simulink model "Modelo_Respiratorio"  (R2018a)
settings: Solver=FixedStepAuto  StartTime=0.0  StopTime=15  FixedStep=0.01  MaxStep=0.05  RelTol=1e-3  AbsTol=1e-3
model workspace (MAT data in the model file):
  FR = Simulink.Parameter
  FR.Value = Simulink.data.Expression
  FR.Value.ExpressionString = "FR"
  FR.DataType = 'auto'
  FR.Dimensions = -1
values from neighbouring files (symbols this model uses):
  a = str2num(get(handles.FR, 'String'))    [Ventiladorcito.m]
  b = str2num(get(handles.PEEP, 'String'))    [Ventiladorcito.m]
  c = str2num(get(handles.PP, 'String'))    [Ventiladorcito.m]
  d = round(1/(d+1),2)*100    [Ventiladorcito.m]
  f = str2num(get(handles.CL, 'String'))    [Ventiladorcito.m]
  g = str2num(get(handles.Cw, 'String'))    [Ventiladorcito.m]
  h = str2num(get(handles.Rc, 'String'))    [Ventiladorcito.m]
  j = str2num(get(handles.Rp, 'String'))    [Ventiladorcito.m]
  k = str2num(get(handles.Cs, 'String'))    [Ventiladorcito.m]
settings Model: Creator=Biomecanica  LastModifiedBy=David
settings SolverCC: AutoScaleAbsTol=off
settings DataIOCC: SaveFormat=Array  SignalLoggingSaveFormat=ModelDataLogs  SaveOutput=off  SaveTime=off
settings OptimizationCC: BlockReduction=off  BooleanDataType=off  LifeSpan=inf
settings DebuggingCC: SaveWithParameterizedLinksMsg=none  UnderspecifiedInitializationDetection=Classic  MergeDetectMultiDrivingBlocksExec=none  SignalResolutionControl=TryResolveAllWithWarning  MultiTaskDSMMsg=warning  MultiTaskCondExecSysMsg=none  SFUnexpectedBacktrackingDiag=warning  SFNoUnconditionalDefaultTransitionDiag=warning  SFExecutionAtInitializationDiag=none
settings HardwareCC: TargetUnknown=on
settings ModelReferenceCC: PropagateSignalLabelsOutOfModel=off
settings RTWCC: TemplateMakefile=grt_vc.tmf
settings CodeAppCC: StateflowObjectComments=on
settings GRTTargetCC: TargetLangStandard=C89/C90 (ANSI)  CombineOutputUpdateFcns=off  GRTInterface=on
settings ConfigComp: CovMetricSettings=dw  CovHtmlReporting=on  CovSaveCumulativeToWorkspaceVar=on  CovSaveSingleToWorkspaceVar=on  CovExternalEMLEnable=off

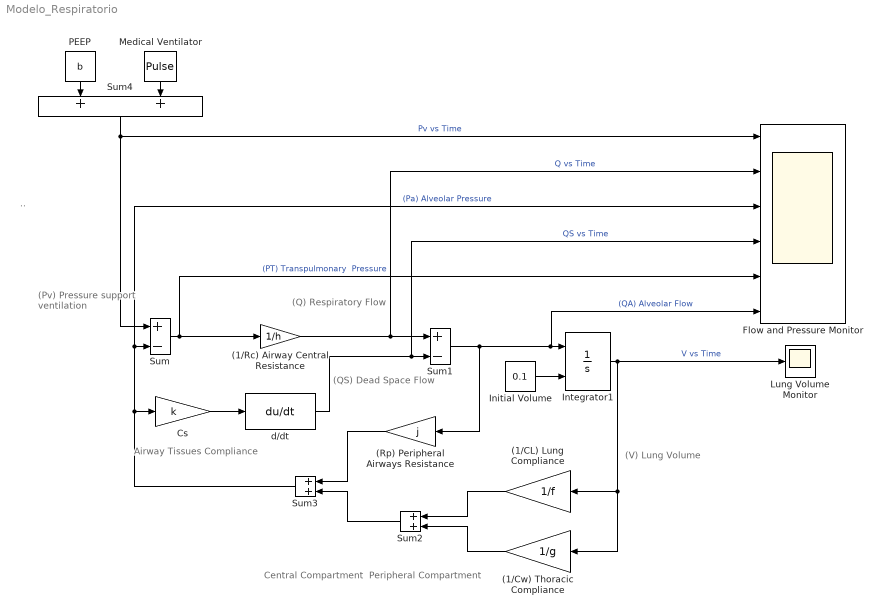
== system Modelo_Respiratorio ==
  note: Airway Tissues
      | Compliance
  note: ..
  note: Peripheral
      | Compartment
  note: (Pv)
      | Pressure support ventilation
  note: (Q)
      | Respiratory
      | Flow
  note: (V)
      | Lung Volume
  note: (QS)
      | Dead Space
      | Flow
  note: Central
      | Compartment
  " Medical Ventilator" : DiscretePulseGenerator  PulseType=Time based  Amplitude=c  Period=60/a  PulseWidth=d
  (1/CL) Lung Compliance : Gain  Gain=1/f  SaturateOnIntegerOverflow=on  OutDataTypeStr=Inherit: Same as input  ParamDataTypeStr=Inherit: Same as input
  (1/Cw) Thoracic Compliance : Gain  Gain=1/g  SaturateOnIntegerOverflow=on  OutDataTypeStr=Inherit: Same as input  ParamDataTypeStr=Inherit: Same as input
  "(1/Rc) Airway Central Resistance " : Gain  Gain=1/h  SaturateOnIntegerOverflow=on  OutDataTypeStr=Inherit: Same as input  ParamDataTypeStr=Inherit: Same as input
  "(Rp) Peripheral Airways Resistance " : Gain  Gain=j  SaturateOnIntegerOverflow=on  OutDataTypeStr=Inherit: Same as input  ParamDataTypeStr=Inherit: Same as input
  "Cs " : Gain  Gain=k  SaturateOnIntegerOverflow=on  OutDataTypeStr=Inherit: Same as input  ParamDataTypeStr=Inherit: Same as input
  Flow and Pressure Monitor : Scope  NumInputPorts=6
  Initial Volume : Constant  Value=0.1
  Integrator1 : Integrator  InitialConditionSource=external
  Lung Volume Monitor : Scope
  PEEP : Constant  Value=b
  Sum : Sum  Inputs=+-  SaturateOnIntegerOverflow=on  InputSameDT=on  OutDataTypeStr=Inherit: Same as first input
  Sum1 : Sum  Inputs=+-  SaturateOnIntegerOverflow=on  InputSameDT=on  OutDataTypeStr=Inherit: Same as first input
  Sum2 : Sum  SaturateOnIntegerOverflow=on  InputSameDT=on  OutDataTypeStr=Inherit: Same as first input
  Sum3 : Sum  SaturateOnIntegerOverflow=on  InputSameDT=on  OutDataTypeStr=Inherit: Same as first input
  Sum4 : Sum  SaturateOnIntegerOverflow=on  InputSameDT=on  OutDataTypeStr=Inherit: Same as first input
  "d/dt " : Derivative  CoefficientInTFapproximation=1
  wires:
  Sum/1 -> "(1/Rc) Airway Central Resistance "/1, Flow and Pressure Monitor/5  "(PT) Transpulmonary  Pressure"
  "(1/Rc) Airway Central Resistance "/1 -> Sum1/1, Flow and Pressure Monitor/2  "Q vs Time"
  "Cs "/1 -> "d/dt "/1
  "d/dt "/1 -> Flow and Pressure Monitor/4, Sum1/2  "QS vs Time"
  (1/CL) Lung Compliance/1 -> Sum2/1
  (1/Cw) Thoracic Compliance/1 -> Sum2/2
  Integrator1/1 -> Lung Volume Monitor/1, (1/CL) Lung Compliance/1, (1/Cw) Thoracic Compliance/1  "V vs Time"
  "(Rp) Peripheral Airways Resistance "/1 -> Sum3/1
  Sum2/1 -> Sum3/2
  Sum1/1 -> Flow and Pressure Monitor/6, Integrator1/1, "(Rp) Peripheral Airways Resistance "/1  "(QA) Alveolar Flow"
  Sum3/1 -> "Cs "/1, Flow and Pressure Monitor/3, Sum/2  "(Pa) Alveolar Pressure"
  Initial Volume/1 -> Integrator1/2
  Sum4/1 -> Flow and Pressure Monitor/1, Sum/1  "Pv vs Time"
  " Medical Ventilator"/1 -> Sum4/2
  PEEP/1 -> Sum4/1
